simulink model "TenzoDecV3DeltaP"  (Simulink 7.9)
settings: Solver=ode23s  StartTime=0.0  StopTime=15  RelTol=1e-3
values from neighbouring files (symbols this model uses):
  AMI = AK1    [DecV3Vars.m]
  AMin = [ ... (first row only)    [DecV3Vars.m]
  Aoss = AMin-V*ClocalMin    [DecV3Vars.m]
  BMI = BK1    [DecV3Vars.m]
  Bmod = [M BMin]    [DecV3Vars.m]
  Boss = [BMin-V*D V M-V*N]    [DecV3Vars.m]
  ClocalMin = [ ... (first row only)    [DecV3Vars.m]
  CMI = eye(q*mu)    [DecV3Vars.m]
  Coss = eye(n)    [DecV3Vars.m]
  D_phi = [1 1877.59274550691 0]    [DecV3Vars.m]
  D_psi = [1 1877.59274550691 0]    [DecV3Vars.m]
  D_theta = [1 1877.59274550691 0]    [DecV3Vars.m]
  D_thrust = [1 5043.9968441748 6107158.06951568]    [DecV3Vars.m]
  DMI = zeros(q*mu,q)    [DecV3Vars.m]
  Dmod = [N D]    [DecV3Vars.m]
  Doss = zeros(size(Boss))    [DecV3Vars.m]
  EasyHardSat = 0    [DecV3Vars.m]
  F1 = F(:,size(AMin,1)+1:size(F,2))    [DecV3Vars.m]
  F2 = F(:,1:size(AMin,1))    [DecV3Vars.m]
  k1 = 1    [DecV3Vars.m]
  k2 = 1.869    [DecV3Vars.m]
  k3 = 2.002    [DecV3Vars.m]
  k4 = 1.996    [DecV3Vars.m]
  Kt = ct*rho*rp^2*pi()    [DecV3Vars.m]
  Ktm = Km/Kt    [DecV3Vars.m]
  lx = 28.8e-3    (= 0.0288)    [DecV3Vars.m]
  ly = 28.8e-3    (= 0.0288)    [DecV3Vars.m]
  N_phi = [3029.1617545382 41884.8274476077 0]    [DecV3Vars.m]
  N_psi = [3029.1617545382 41884.8274476077 0]    [DecV3Vars.m]
  N_theta = [3029.1617545382 41884.8274476077 0]    [DecV3Vars.m]
  N_thrust = [1073231686.12918 1273486031.3238]    [DecV3Vars.m]
  omega = 0.5    [DecV3Vars.m]
  satMaxRPM = 6000    [DecV3Vars.m]
  satMinRPM = -1300    [DecV3Vars.m]
  satNegThrust = 6    [DecV3Vars.m]
  satTau = 100    [DecV3Vars.m]
  satThrust = 56    [DecV3Vars.m]
  tc = 0.0436    [DecV3Vars.m]
undefined symbols (not defined in the file or in its folder): magnitude, sigbuilder_block
libraries: simulink x6
settings Model: Creator=danilo  LastModifiedBy=userk
settings DebuggingCC: FcnCallInpInsideContextMsg=Use local settings
settings GRTTargetCC: CombineOutputUpdateFcns=off  GRTInterface=on

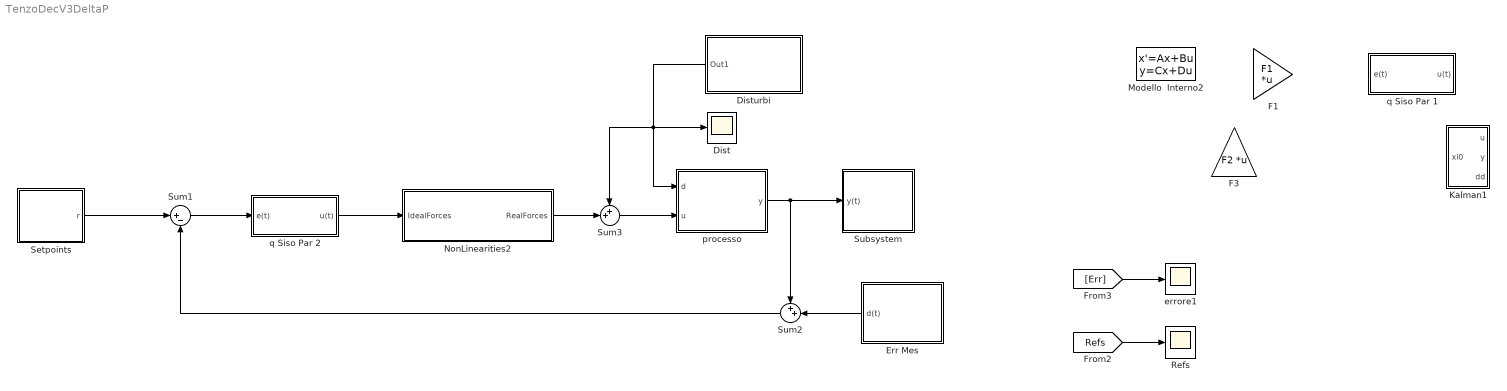
== system TenzoDecV3DeltaP ==
  Dist : Scope
      settings: TimeRange=15  YMin=-0.1  YMax=0.09  SaveName=ScopeData22
  Disturbi : Subsystem
  Err Mes : Subsystem
  F1 : Gain  Gain=F1  Multiplication=Matrix(K*u) (u vector)
  F3 : Gain  Gain=F2  Multiplication=Matrix(K*u) (u vector)
  Kalman1 : Subsystem
  Modello  Interno2 : StateSpace  A=AMI  B=BMI  C=CMI  D=DMI
  NonLinearities2 : Subsystem
  Refs : Scope
  Setpoints : Subsystem
  Subsystem : Subsystem
  Sum1 : Sum  Inputs=|+-
  Sum2 : Sum  Inputs=++|
  Sum3 : Sum  Inputs=++|
  errore1 : Scope
      settings: SaveName=ScopeData8
  processo : Subsystem
  q Siso Par 1 : Subsystem
  q Siso Par 2 : Subsystem
  wires:
  Setpoints/1(r) -> Sum1/1
  processo/1(y) -> Sum2/1, Subsystem/1(y(t))
  Sum1/1 -> q Siso Par 2/1(e(t))
  [Refs] -> Refs/1
  [Err] -> errore1/1
  q Siso Par 2/1(u(t)) -> NonLinearities2/1(IdealForces)
  NonLinearities2/1(RealForces) -> Sum3/2
  Err Mes/1("  d(t)") -> Sum2/2
  Sum2/1 -> Sum1/2
  Disturbi/1(Out1) -> processo/1(d), Dist/1, Sum3/1
  Sum3/1 -> processo/2(u)

== system TenzoDecV3DeltaP/Disturbi ==
  Disturbi Hard : Subsystem
  DisturboEasy : Subsystem
  Manual Switch : simulink/Signal Routing/Manual Switch  sw=0  action=0  varsize=off
  Out1 : Outport
  wires:
  DisturboEasy/1(Out1) -> Manual Switch/1
  Disturbi Hard/1("  d(t)") -> Manual Switch/2
  Manual Switch/1 -> Out1/1

== system TenzoDecV3DeltaP/Err Mes ==
  0.03 sen(80t) : Sin  Amplitude=0.003  Frequency=80  Phase=1  SampleTime=0
  0.2 sen(0.5 t) : Sin  Amplitude=0.02  Frequency=50  Phase=1  SampleTime=0
  Gain : Gain
  Manual Switch1 : simulink/Signal Routing/Manual Switch  sw=0  action=0  varsize=off
  P(s)1 : TransferFcn  Numerator=1  Denominator=[1 9]
  Scope2 : Scope
      settings: SaveName=ScopeData21
  Sum3 : Sum
  Uniform Random Number : UniformRandomNumber  Minimum=-0.05  Maximum=0.05  SampleTime=0.1
  "  d(t)" : Outport
  wires:
  Uniform Random Number/1 -> Sum3/1
  0.2 sen(0.5 t)/1 -> Sum3/2
  Sum3/1 -> P(s)1/1
  0.03 sen(80t)/1 -> Manual Switch1/1
  P(s)1/1 -> Manual Switch1/2
  Gain/1 -> "  d(t)"/1, Scope2/1
  Manual Switch1/1 -> Gain/1

== system TenzoDecV3DeltaP/Kalman1 ==
  u : Inport
  y : Inport  Port=2
  dd : Inport  Port=3
  Mux : Mux  Inputs=[4 4 1]
  filtro di kalman : StateSpace  A=Aoss  B=Boss  C=Coss  D=Doss
  xi0 : Outport
  wires:
  dd/1 -> Mux/3
  y/1 -> Mux/2
  filtro di kalman/1 -> xi0/1
  u/1 -> Mux/1
  Mux/1 -> filtro di kalman/1

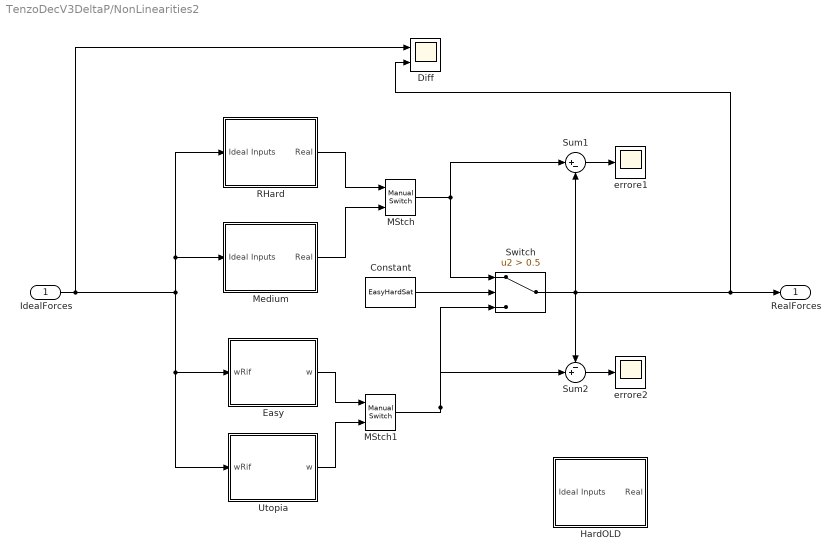
== system TenzoDecV3DeltaP/NonLinearities2 ==
  IdealForces : Inport
  Constant : Constant  Value=EasyHardSat
  Diff : Scope  NumInputPorts=2
      settings: YMin=-37.5~-37.5  YMax=12.5~12.5  SaveName=ScopeData3
  Easy : Subsystem
  HardOLD : Subsystem
  MStch : simulink/Signal Routing/Manual Switch  sw=0  action=0  varsize=off
  MStch1 : simulink/Signal Routing/Manual Switch  sw=1  action=0  varsize=off
  Medium : Subsystem
  RHard : Subsystem
  Sum1 : Sum  Inputs=|+-
  Sum2 : Sum  Inputs=-+|
  Switch : Switch  Criteria=u2 > Threshold  Threshold=0.5
  Utopia : Subsystem
  errore1 : Scope
      settings: SaveName=ScopeData18
  errore2 : Scope
      settings: SaveName=ScopeData20
  RealForces : Outport
  wires:
  Sum2/1 -> errore2/1
  Sum1/1 -> errore1/1
  IdealForces/1 -> Medium/1(Ideal Inputs), RHard/1(Ideal Inputs), Easy/1(wRif), Utopia/1(wRif), Diff/1
  Switch/1 -> Sum2/1, Sum1/2, RealForces/1, Diff/2
  Constant/1 -> Switch/2
  MStch/1 -> Switch/1, Sum1/1
  RHard/1(Real) -> MStch/1
  Medium/1(Real) -> MStch/2
  MStch1/1 -> Switch/3, Sum2/2
  Easy/1(w) -> MStch1/1
  Utopia/1(w) -> MStch1/2

== system TenzoDecV3DeltaP/Setpoints ==
  Mux : Mux  Inputs=[1 1 1 1]
  PsiRef : Step  Time=0.8  After=2.5  SampleTime=0
  Signal Builder : Subsystem  Tag=STV Subsys  LoadFcn=sigbuilder_block('load');  StartFcn=sigbuilder_block('start');  StopFcn=sigbuilder_block('stop');  ClipboardFcn=sigbuilder_block('clipboard');  mask(Sigbuilder block){}
      mask help: Simulink:masks:SigbuilderBlock_MD
      mask init:
      | if ~strcmp(get_param(bdroot(gcbh),'SimulationStatus'),'stopped') tuvar = sigbuilder_block('maskInit'); end
      settings: CopyFcn=sigbuilder_block('copy');  DeleteFcn=sigbuilder_block('delete');  ModelCloseFcn=sigbuilder_block('modelClose');  PreSaveFcn=sigbuilder_block('preSave');  PauseFcn=sigbuilder_block('pause');  ContinueFcn=sigbuilder_block('continue');  NameChangeFcn=sigbuilder_block('namechange');  OpenFcn=sigbuilder_block('open',[357.6 120.8 550.4 400 ]);  CloseFcn=sigbuilder_block('close');
      mask Display: plot(0, 0, 100, 100,[2, 2, 32, 32, 2], [68, 8, 8, 68, 68],[32, 2], [38, 38], [32, 19, 2],[53, 60, 44], [32, 17, 17, 2],[16, 16, 31, 31]);txt = getActiveGroup(gcbh);text(2, 100, txt,'verticalAlignment', 'top');
  ThetRef : Step  Time=0.5  After=2  SampleTime=0
  phiRef : Step  After=1.5  SampleTime=0
  r : Outport
  tag scope: Refs=global
  wires:
  Mux/1 -> r/1, [Refs]
  phiRef/1 -> Mux/1
  ThetRef/1 -> Mux/2
  PsiRef/1 -> Mux/3
  Signal Builder/1(Signal 1) -> Mux/4

== system TenzoDecV3DeltaP/Subsystem ==
  y(t) : Inport
  Output : Subsystem
  uscite : Scope
      settings: TimeRange=15  YMin=-1.4e+10  YMax=6e+09  SaveName=ScopeData2
  wires:
  [Refs] -> Output/2(In2)
  y(t)/1 -> Output/1(In1), uscite/1

== system TenzoDecV3DeltaP/processo ==
  d : Inport
  u : Inport  Port=2
  Mux : Mux  Inputs=[1 4]
  Processo1 : StateSpace  A=AMin  B=Bmod  C=ClocalMin  D=Dmod
  y : Outport
  wires:
  Mux/1 -> Processo1/1
  d/1 -> Mux/1
  Processo1/1 -> y/1
  u/1 -> Mux/2

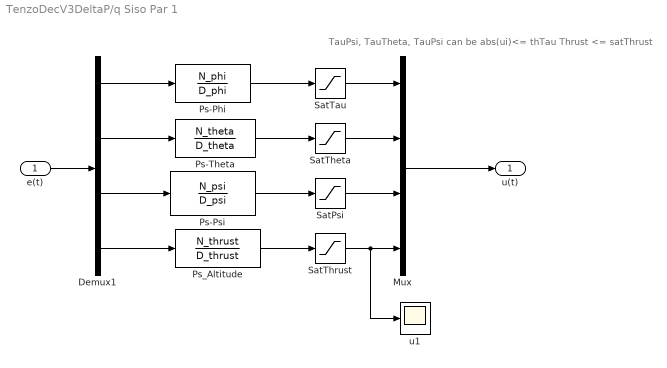
== system TenzoDecV3DeltaP/q Siso Par 1 ==
  note: TauPsi, TauTheta, TauPsi
      |  can be abs(ui)<= thTau
      | Thrust <= satThrust
  e(t) : Inport
  Demux1 : Demux
  Mux : Mux
  Ps-Phi : TransferFcn  Numerator=N_phi  Denominator=D_phi
  Ps-Psi : TransferFcn  Numerator=N_psi  Denominator=D_psi
  Ps-Theta : TransferFcn  Numerator=N_theta  Denominator=D_theta
  Ps_Altitude : TransferFcn  Numerator=N_thrust  Denominator=D_thrust
  SatPsi : Saturate  UpperLimit=satTau  LowerLimit=-satTau
  SatTau : Saturate  UpperLimit=satTau  LowerLimit=-satTau
  SatTheta : Saturate  UpperLimit=satTau  LowerLimit=-satTau
  SatThrust : Saturate  UpperLimit=satThrust  LowerLimit=-satNegThrust
  u1 : Scope
      settings: SaveName=ScopeData9
  u(t) : Outport
  wires:
  SatTau/1 -> Mux/1
  SatTheta/1 -> Mux/2
  SatPsi/1 -> Mux/3
  SatThrust/1 -> u1/1, Mux/4
  Demux1/1 -> Ps-Phi/1
  Demux1/3 -> Ps-Psi/1
  Demux1/4 -> Ps_Altitude/1
  Ps-Phi/1 -> SatTau/1
  Ps_Altitude/1 -> SatThrust/1
  Demux1/2 -> Ps-Theta/1
  Ps-Theta/1 -> SatTheta/1
  Ps-Psi/1 -> SatPsi/1
  e(t)/1 -> Demux1/1
  Mux/1 -> u(t)/1

== system TenzoDecV3DeltaP/q Siso Par 2 ==
  note: TauPsi, TauTheta, TauPsi
      |  can be abs(ui)<= thTau
      | Thrust <= satThrust
  e(t) : Inport
  Demux1 : Demux
  Mux : Mux
  Old q SISO + sat : Subsystem
  Ps-Phi : TransferFcn  Numerator=N_phi  Denominator=D_phi
  Ps-Psi : TransferFcn  Numerator=N_psi  Denominator=D_psi
  Ps-Theta : TransferFcn  Numerator=N_theta  Denominator=D_theta
  Ps_Altitude : TransferFcn  Numerator=N_thrust  Denominator=D_thrust
  To Workspace : ToWorkspace  VariableName=simout  SampleTime=-1  SaveFormat=Structure
  u1 : Scope
      settings: YMin=-8e+08  YMax=5e+07  SaveName=ScopeData9
  u(t) : Outport
  wires:
  Mux/1 -> u(t)/1
  e(t)/1 -> Demux1/1, To Workspace/1, [Err]
  Ps-Psi/1 -> Mux/3
  Ps-Theta/1 -> Mux/2
  Demux1/2 -> Ps-Theta/1
  Ps_Altitude/1 -> Mux/4, u1/1
  Ps-Phi/1 -> Mux/1
  Demux1/4 -> Ps_Altitude/1
  Demux1/3 -> Ps-Psi/1
  Demux1/1 -> Ps-Phi/1

== system TenzoDecV3DeltaP/Disturbi/Disturbi Hard ==
  0.2 sen(0.5 t) : Sin  Amplitude=0.2  Frequency=0.5  Phase=1  SampleTime=0
  0.2 sen(0.5 t)1 : Sin  Amplitude=0.1  Frequency=1.5  Phase=1.5  SampleTime=0
  0.5sen(0.5 t) : Sin  Amplitude=0.5  Frequency=0.5  Phase=1  SampleTime=0
  Manual Switch1 : simulink/Signal Routing/Manual Switch  sw=0  action=0  varsize=off
  P(s)1 : TransferFcn  Numerator=1  Denominator=[1 4]
  Sum3 : Sum  Inputs=+++
  Uniform Random Number : UniformRandomNumber  Minimum=-0.5  Maximum=0.5  SampleTime=0.1
  d(t) : Gain
  d(t) raw : Scope
      settings: TimeRange=15  YMin=-0.65  YMax=0.05  SaveName=ScopeData24
  "  d(t)" : Outport
  wires:
  Uniform Random Number/1 -> Sum3/1
  0.2 sen(0.5 t)/1 -> Sum3/3
  Sum3/1 -> P(s)1/1, d(t) raw/1
  0.5sen(0.5 t)/1 -> Manual Switch1/1
  P(s)1/1 -> Manual Switch1/2
  d(t)/1 -> "  d(t)"/1
  Manual Switch1/1 -> d(t)/1
  0.2 sen(0.5 t)1/1 -> Sum3/2

== system TenzoDecV3DeltaP/Disturbi/DisturboEasy ==
  Clock : Clock
  Constant : Constant  Value=0
  Constant1 : Constant  Value=0
  Manual Switch : simulink/Signal Routing/Manual Switch  sw=0  action=0  varsize=off
  Switch : Switch  Threshold=5
  dist : Scope
      settings: SaveName=ScopeData5
  disturbo : Subsystem
  Out1 : Outport
  wires:
  Clock/1 -> Switch/2
  disturbo/1(d) -> Switch/1
  Constant/1 -> Switch/3
  Constant1/1 -> Manual Switch/1
  Switch/1 -> Manual Switch/2
  Manual Switch/1 -> dist/1, Out1/1

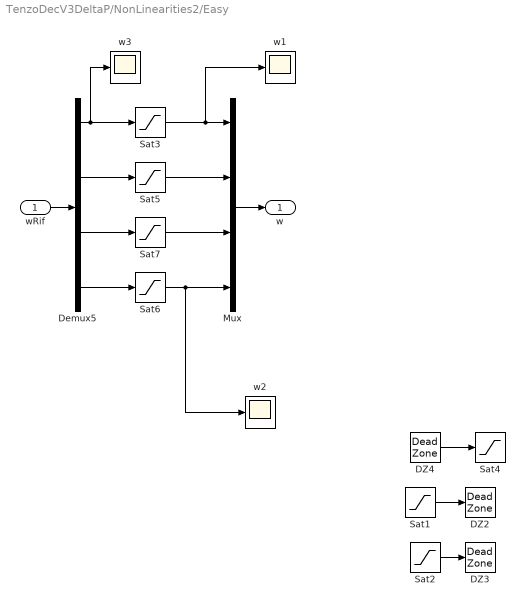
== system TenzoDecV3DeltaP/NonLinearities2/Easy ==
  wRif : Inport
  DZ2 : DeadZone  LowerValue=0  UpperValue=deadMotorsZone  SaturateOnIntegerOverflow=on
  DZ3 : DeadZone  LowerValue=0  UpperValue=deadMotorsZone  SaturateOnIntegerOverflow=on
  DZ4 : DeadZone  LowerValue=0  UpperValue=deadMotorsZone  SaturateOnIntegerOverflow=on
  Demux5 : Demux
  Mux : Mux
  Sat1 : Saturate  UpperLimit=satMaxRPM  LowerLimit=0
  Sat2 : Saturate  UpperLimit=satMaxRPM  LowerLimit=0
  Sat3 : Saturate  UpperLimit=satTau  LowerLimit=-satTau
  Sat4 : Saturate  UpperLimit=satMaxRPM  LowerLimit=0
  Sat5 : Saturate  UpperLimit=satTau  LowerLimit=-satTau
  Sat6 : Saturate  UpperLimit=satThrust  LowerLimit=-satNegThrust
  Sat7 : Saturate  UpperLimit=satTau  LowerLimit=-satTau
  w1 : Scope
      settings: YMin=-1.5e+42  YMax=2.25e+42  SaveName=ScopeData15
  w2 : Scope
      settings: YMin=-8e+50  YMax=5e+50  SaveName=ScopeData10
  w3 : Scope
      settings: YMin=904.495  YMax=999.705  SaveName=ScopeData16
  w : Outport
  wires:
  Demux5/4 -> Sat6/1
  Demux5/3 -> Sat7/1
  Demux5/2 -> Sat5/1
  Sat7/1 -> Mux/3
  Sat6/1 -> w2/1, Mux/4
  Sat5/1 -> Mux/2
  Sat3/1 -> Mux/1, w1/1
  Demux5/1 -> Sat3/1, w3/1
  wRif/1 -> Demux5/1
  Mux/1 -> w/1
  DZ4/1 -> Sat4/1
  Sat1/1 -> DZ2/1
  Sat2/1 -> DZ3/1

== system TenzoDecV3DeltaP/NonLinearities2/HardOLD ==
  Ideal Inputs : Inport
  Demux11 : Demux
  Motors : Subsystem
  Mux3 : Mux
  T*toW : MATLAB Function  TreatAsAtomicUnit=on
  WtoTreal : Subsystem
  ideal : Scope
      settings: YMin=-5e+71  YMax=4e+71  SaveName=ScopeData25
  real : Scope
      settings: YMin=-2.5e+113  YMax=4.25e+114  SaveName=ScopeData26
  wReal : Scope
      settings: SaveName=ScopeData27
  wideal : Scope
      settings: YMin=-4.5e+73  YMax=4.5e+73  SaveName=ScopeData23
  Real : Outport
  wires:
  WtoTreal/1(U(t)) -> real/1, Real/1
  Ideal Inputs/1 -> ideal/1, Demux11/1
  Mux3/1 -> wideal/1, Motors/1(wRif)
  Motors/1(w) -> wReal/1, WtoTreal/1(w(t))
  Demux11/1 -> T*toW/1(taux)
  Demux11/2 -> T*toW/2(tauy)
  Demux11/3 -> T*toW/3(tauz)
  Demux11/4 -> T*toW/4(Thrust)
  T*toW/1(w1) -> Mux3/1
  T*toW/2(w2) -> Mux3/2
  T*toW/3(w3) -> Mux3/3
  T*toW/4(w4) -> Mux3/4

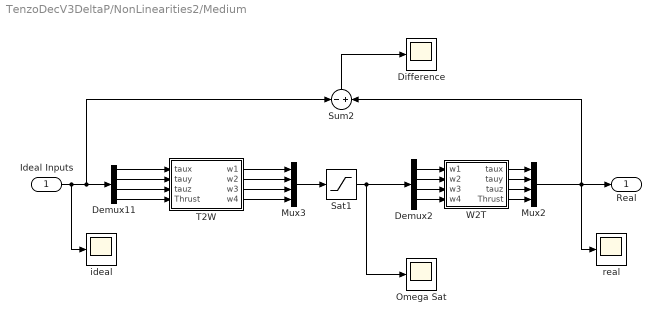
== system TenzoDecV3DeltaP/NonLinearities2/Medium ==
  Ideal Inputs : Inport
  Demux11 : Demux
  Demux2 : Demux
  Difference : Scope
      settings: YMin=-4e-08  YMax=1.2e-07  SaveName=ScopeData28
  Mux2 : Mux
  Mux3 : Mux
  Omega Sat : Scope
      settings: YMin=-6000  YMax=6000  SaveName=ScopeData29
  Sat1 : Saturate  UpperLimit=8000  LowerLimit=-10000
  Sum2 : Sum  Inputs=-+
  T2W : MATLAB Function  TreatAsAtomicUnit=on
  W2T : MATLAB Function  TreatAsAtomicUnit=on
  ideal : Scope
      settings: YMin=-5e+71  YMax=4e+71  SaveName=ScopeData25
  real : Scope
      settings: YMin=-2.5e+113  YMax=4.25e+114  SaveName=ScopeData26
  Real : Outport
  wires:
  T2W/4(w4) -> Mux3/4
  T2W/3(w3) -> Mux3/3
  T2W/2(w2) -> Mux3/2
  T2W/1(w1) -> Mux3/1
  Demux11/4 -> T2W/4(Thrust)
  Demux11/3 -> T2W/3(tauz)
  Demux11/2 -> T2W/2(tauy)
  Demux11/1 -> T2W/1(taux)
  Mux3/1 -> Sat1/1
  Ideal Inputs/1 -> ideal/1, Demux11/1, Sum2/1
  Mux2/1 -> real/1, Real/1, Sum2/2
  Demux2/1 -> W2T/1(w1)
  Demux2/2 -> W2T/2(w2)
  Demux2/3 -> W2T/3(w3)
  Demux2/4 -> W2T/4(w4)
  W2T/1(taux) -> Mux2/1
  W2T/2(tauy) -> Mux2/2
  W2T/3(tauz) -> Mux2/3
  W2T/4(Thrust) -> Mux2/4
  Sum2/1 -> Difference/1
  Sat1/1 -> Demux2/1, Omega Sat/1

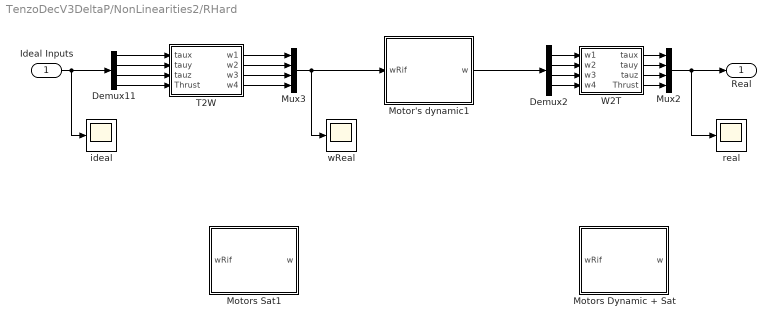
== system TenzoDecV3DeltaP/NonLinearities2/RHard ==
  Ideal Inputs : Inport
  Demux11 : Demux
  Demux2 : Demux
  Motor's dynamic1 : Subsystem
  Motors Dynamic + Sat : Subsystem
  Motors Sat1 : Subsystem
  Mux2 : Mux
  Mux3 : Mux
  T2W : MATLAB Function  TreatAsAtomicUnit=on
  W2T : MATLAB Function  TreatAsAtomicUnit=on
  ideal : Scope
      settings: YMin=-5e+71  YMax=4e+71  SaveName=ScopeData25
  real : Scope
      settings: YMin=-2.5e+113  YMax=4.25e+114  SaveName=ScopeData26
  wReal : Scope
      settings: YMin=-7500  YMax=35000  SaveName=ScopeData27
  Real : Outport
  wires:
  W2T/4(Thrust) -> Mux2/4
  W2T/3(tauz) -> Mux2/3
  W2T/2(tauy) -> Mux2/2
  W2T/1(taux) -> Mux2/1
  Demux2/4 -> W2T/4(w4)
  Demux2/3 -> W2T/3(w3)
  Demux2/2 -> W2T/2(w2)
  Demux2/1 -> W2T/1(w1)
  Mux2/1 -> Real/1, real/1
  Ideal Inputs/1 -> Demux11/1, ideal/1
  Mux3/1 -> wReal/1, Motor's dynamic1/1(wRif)
  Demux11/1 -> T2W/1(taux)
  Demux11/2 -> T2W/2(tauy)
  Demux11/3 -> T2W/3(tauz)
  Demux11/4 -> T2W/4(Thrust)
  T2W/1(w1) -> Mux3/1
  T2W/2(w2) -> Mux3/2
  T2W/3(w3) -> Mux3/3
  T2W/4(w4) -> Mux3/4
  Motor's dynamic1/1(w) -> Demux2/1

== system TenzoDecV3DeltaP/NonLinearities2/Utopia ==
  wRif : Inport
  DZ3 : DeadZone  LowerValue=0  UpperValue=deadMotorsZone  SaturateOnIntegerOverflow=on
  Demux5 : Demux
  Mux : Mux
  Sat2 : Saturate  UpperLimit=satMaxRPM  LowerLimit=0
  w : Outport
  wires:
  Sat2/1 -> DZ3/1
  ? -> ?
  Mux/1 -> w/1
  wRif/1 -> Demux5/1
  Demux5/1 -> Mux/1
  Demux5/2 -> Mux/2
  Demux5/3 -> Mux/3
  Demux5/4 -> Mux/4

== system TenzoDecV3DeltaP/Setpoints/Signal Builder ==
  Demux : Demux  Tag=STV Demux  Outputs=1
  FromWs : FromWorkspace  Tag=STV FromWs  VariableName=tuvar  SampleTime=0  SigBuilderData=DataTag0  VnvData=DataTag1
      SigBuilderData=|
      | common.afterFinalStr = 'Extrapolate'
      | common.sampleTime = 0
      | dataSet.timeRange = [0 10]
      | dataSet.name = 'Group 1'
      | sbobj.Groups.Name = 'Group 1'
      | sbobj.Groups.Signals.Name = 'Signal 1'
      | sbobj.Groups.Signals.XData = [0 4.06 6 6 10]
      | sbobj.Groups.Signals.YData = [-2.77555756156e-17 1 1 0.995 0.795]
  Signal 1 : Outport  Tag=STV Outport
  wires:
  Demux/1 -> Signal 1/1
  FromWs/1 -> Demux/1

== system TenzoDecV3DeltaP/Subsystem/Output ==
  In1 : Inport
  In2 : Inport  Port=2
  Demux1 : Demux
  Demux2 : Demux
  Mux{2..5} (4 alike) : Mux  Inputs=2
  uscite{,1..3} (4 alike) : Scope
      uscite settings: TickLabels=on  YMin=1.495  YMax=1.5065
      uscite1 settings: TickLabels=on  TimeRange=30  YMin=0.75  YMax=4.25  SaveName=ScopeData4
      uscite2 settings: TickLabels=on  TimeRange=15  YMin=-1.75e+15  YMax=1.75e+15  SaveName=ScopeData6
      uscite3 settings: TickLabels=on  YMin=0  YMax=1.05  SaveName=ScopeData7
  wires:
  Demux1/1 -> Mux3/2
  In2/1 -> Demux1/1
  In1/1 -> Demux2/1
  Mux3/1 -> uscite/1
  Demux2/1 -> Mux3/1
  Mux2/1 -> uscite1/1
  Demux2/2 -> Mux2/1
  Mux4/1 -> uscite2/1
  Demux2/3 -> Mux4/1
  Mux5/1 -> uscite3/1
  Demux2/4 -> Mux5/1
  Demux1/2 -> Mux2/2
  Demux1/3 -> Mux4/2
  Demux1/4 -> Mux5/2

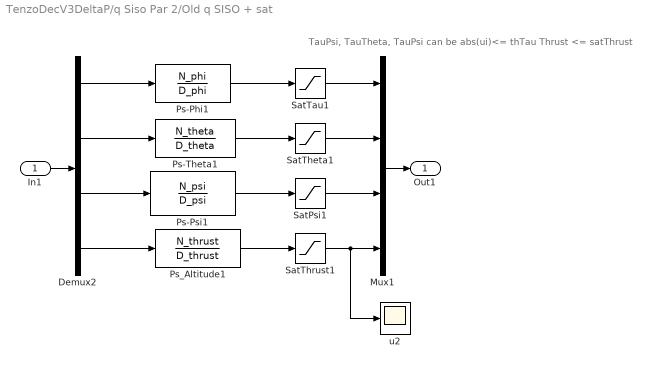
== system TenzoDecV3DeltaP/q Siso Par 2/Old q SISO + sat ==
  note: TauPsi, TauTheta, TauPsi
      |  can be abs(ui)<= thTau
      | Thrust <= satThrust
  In1 : Inport
  Demux2 : Demux
  Mux1 : Mux
  Ps-Phi1 : TransferFcn  Numerator=N_phi  Denominator=D_phi
  Ps-Psi1 : TransferFcn  Numerator=N_psi  Denominator=D_psi
  Ps-Theta1 : TransferFcn  Numerator=N_theta  Denominator=D_theta
  Ps_Altitude1 : TransferFcn  Numerator=N_thrust  Denominator=D_thrust
  SatPsi1 : Saturate  UpperLimit=satTau  LowerLimit=-satTau
  SatTau1 : Saturate  UpperLimit=satTau  LowerLimit=-satTau
  SatTheta1 : Saturate  UpperLimit=satTau  LowerLimit=-satTau
  SatThrust1 : Saturate  UpperLimit=satThrust  LowerLimit=-satNegThrust
  u2 : Scope
      settings: SaveName=ScopeData12
  Out1 : Outport
  wires:
  Ps-Psi1/1 -> SatPsi1/1
  Ps-Theta1/1 -> SatTheta1/1
  Demux2/2 -> Ps-Theta1/1
  Ps_Altitude1/1 -> SatThrust1/1
  Ps-Phi1/1 -> SatTau1/1
  Demux2/4 -> Ps_Altitude1/1
  Demux2/3 -> Ps-Psi1/1
  Demux2/1 -> Ps-Phi1/1
  SatThrust1/1 -> Mux1/4, u2/1
  SatPsi1/1 -> Mux1/3
  SatTheta1/1 -> Mux1/2
  SatTau1/1 -> Mux1/1
  In1/1 -> Demux2/1
  Mux1/1 -> Out1/1

== system TenzoDecV3DeltaP/Disturbi/DisturboEasy/disturbo ==
  Constant : Constant
  Sine Wave : Sin  Amplitude=0.5  Frequency=omega  SampleTime=0
  Sum2 : Sum  Inputs=|++
  d : Outport
  wires:
  Sine Wave/1 -> Sum2/2
  Constant/1 -> Sum2/1
  Sum2/1 -> d/1

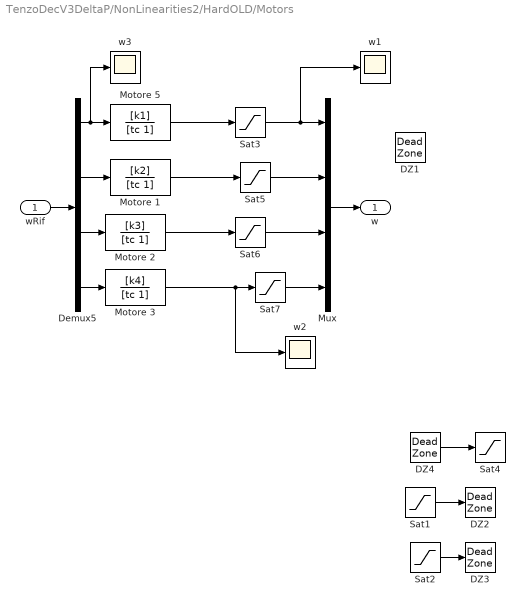
== system TenzoDecV3DeltaP/NonLinearities2/HardOLD/Motors ==
  wRif : Inport
  DZ{1..4} (4 alike) : DeadZone  LowerValue=0  UpperValue=deadMotorsZone  SaturateOnIntegerOverflow=on
  Demux5 : Demux
  Motore 1 : TransferFcn  Numerator=[k2]  Denominator=[tc 1]
  Motore 2 : TransferFcn  Numerator=[k3]  Denominator=[tc 1]
  Motore 3 : TransferFcn  Numerator=[k4]  Denominator=[tc 1]
  Motore 5 : TransferFcn  Numerator=[k1]  Denominator=[tc 1]
  Mux : Mux
  Sat1 : Saturate  UpperLimit=satMaxRPM  LowerLimit=0
  Sat2 : Saturate  UpperLimit=satMaxRPM  LowerLimit=0
  Sat{3,5..7} (4 alike) : Saturate  UpperLimit=satMaxRPM  LowerLimit=satMinRPM
  Sat4 : Saturate  UpperLimit=satMaxRPM  LowerLimit=0
  w1 : Scope
      settings: YMin=-1.5e+42  YMax=2.25e+42  SaveName=ScopeData15
  w2 : Scope
      settings: YMin=-8e+50  YMax=5e+50  SaveName=ScopeData10
  w3 : Scope
      settings: YMin=904.495  YMax=999.705  SaveName=ScopeData16
  w : Outport
  wires:
  Sat7/1 -> Mux/4
  Sat6/1 -> Mux/3
  Sat5/1 -> Mux/2
  Sat3/1 -> w1/1, Mux/1
  Sat2/1 -> DZ3/1
  Sat1/1 -> DZ2/1
  DZ4/1 -> Sat4/1
  Motore 3/1 -> Sat7/1, w2/1
  Motore 2/1 -> Sat6/1
  Motore 1/1 -> Sat5/1
  Motore 5/1 -> Sat3/1
  Mux/1 -> w/1
  wRif/1 -> Demux5/1
  Demux5/4 -> Motore 3/1
  Demux5/3 -> Motore 2/1
  Demux5/2 -> Motore 1/1
  Demux5/1 -> w3/1, Motore 5/1

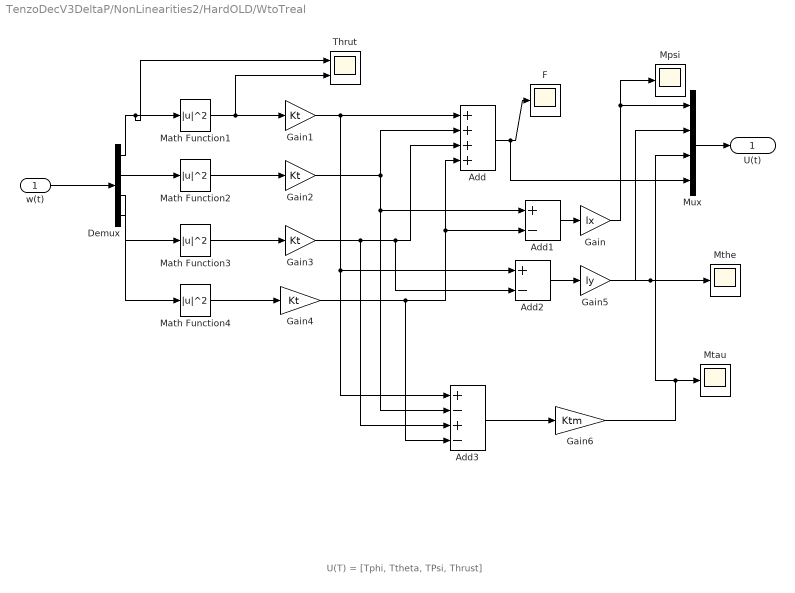
== system TenzoDecV3DeltaP/NonLinearities2/HardOLD/WtoTreal ==
  note: U(T) = [Tphi, Ttheta, TPsi, Thrust]
  w(t) : Inport
  Add : Sum  Inputs=++++
  Add1 : Sum  Inputs=+-
  Add2 : Sum  Inputs=+-
  Add3 : Sum  Inputs=+-+-
  Demux : Demux
  F : Scope
      settings: SaveName=ScopeData17
  Gain : Gain  Gain=lx
  Gain{1..4} (4 alike) : Gain  Gain=Kt
  Gain5 : Gain  Gain=ly
  Gain6 : Gain  Gain=Ktm
  Math Function{1..4} (4 alike) : Math  Operator=magnitude^2  SaturateOnIntegerOverflow=on
  Mpsi : Scope
      settings: SaveName=ScopeData14
  Mtau : Scope
      settings: SaveName=ScopeData11
  Mthe : Scope
      settings: SaveName=ScopeData13
  Mux : Mux
  Thrut : Scope  NumInputPorts=2
      settings: YMin=-5~-5  YMax=5~5  SaveName=ScopeData19
  U(t) : Outport
  wires:
  Math Function1/1 -> Gain1/1, Thrut/2
  Math Function2/1 -> Gain2/1
  Math Function3/1 -> Gain3/1
  Math Function4/1 -> Gain4/1
  Gain1/1 -> Add/1, Add2/1, Add3/1
  Gain2/1 -> Add/2, Add1/1, Add3/2
  Gain3/1 -> Add/3, Add2/2, Add3/3
  Gain4/1 -> Add/4, Add1/2, Add3/4
  Add/1 -> Mux/4, F/1
  Add1/1 -> Gain/1
  Add2/1 -> Gain5/1
  Gain/1 -> Mux/1, Mpsi/1
  Gain5/1 -> Mux/2, Mthe/1
  Add3/1 -> Gain6/1
  Gain6/1 -> Mux/3, Mtau/1
  Demux/1 -> Math Function1/1, Thrut/1
  Demux/2 -> Math Function2/1
  Mux/1 -> U(t)/1
  Demux/3 -> Math Function3/1
  Demux/4 -> Math Function4/1
  w(t)/1 -> Demux/1

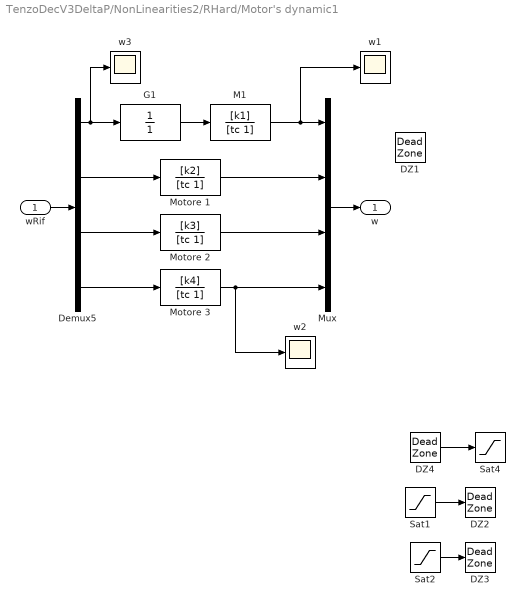
== system TenzoDecV3DeltaP/NonLinearities2/RHard/Motor's dynamic1 ==
  wRif : Inport
  DZ{1..4} (4 alike) : DeadZone  LowerValue=0  UpperValue=deadMotorsZone  SaturateOnIntegerOverflow=on
  Demux5 : Demux
  G1 : TransferFcn  Denominator=[1]
  M1 : TransferFcn  Numerator=[k1]  Denominator=[tc 1]
  Motore 1 : TransferFcn  Numerator=[k2]  Denominator=[tc 1]
  Motore 2 : TransferFcn  Numerator=[k3]  Denominator=[tc 1]
  Motore 3 : TransferFcn  Numerator=[k4]  Denominator=[tc 1]
  Mux : Mux
  Sat1 : Saturate  UpperLimit=satMaxRPM  LowerLimit=0
  Sat2 : Saturate  UpperLimit=satMaxRPM  LowerLimit=0
  Sat4 : Saturate  UpperLimit=satMaxRPM  LowerLimit=0
  w1 : Scope
      settings: YMin=-2250  YMax=3500  SaveName=ScopeData15
  w2 : Scope
      settings: YMin=-8e+50  YMax=5e+50  SaveName=ScopeData10
  w3 : Scope
      settings: YMin=-45000  YMax=60000  SaveName=ScopeData16
  w : Outport
  wires:
  Sat2/1 -> DZ3/1
  Sat1/1 -> DZ2/1
  DZ4/1 -> Sat4/1
  Motore 3/1 -> Mux/4, w2/1
  Motore 2/1 -> Mux/3
  Motore 1/1 -> Mux/2
  G1/1 -> M1/1
  Mux/1 -> w/1
  wRif/1 -> Demux5/1
  Demux5/4 -> Motore 3/1
  Demux5/3 -> Motore 2/1
  Demux5/2 -> Motore 1/1
  Demux5/1 -> w3/1, G1/1
  M1/1 -> w1/1, Mux/1

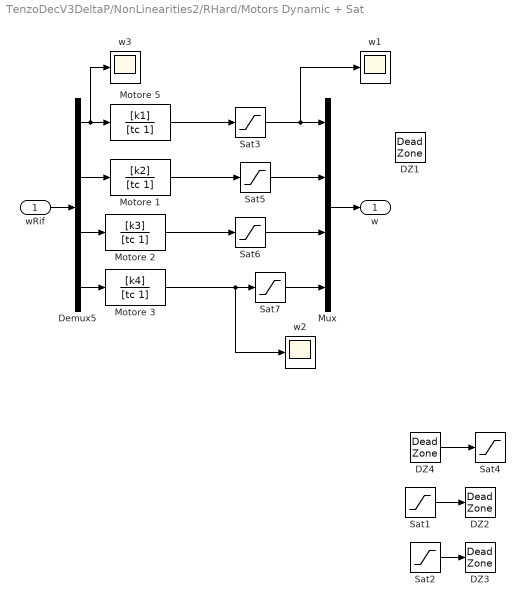
== system TenzoDecV3DeltaP/NonLinearities2/RHard/Motors Dynamic + Sat ==
  wRif : Inport
  DZ{1..4} (4 alike) : DeadZone  LowerValue=0  UpperValue=deadMotorsZone  SaturateOnIntegerOverflow=on
  Demux5 : Demux
  Motore 1 : TransferFcn  Numerator=[k2]  Denominator=[tc 1]
  Motore 2 : TransferFcn  Numerator=[k3]  Denominator=[tc 1]
  Motore 3 : TransferFcn  Numerator=[k4]  Denominator=[tc 1]
  Motore 5 : TransferFcn  Numerator=[k1]  Denominator=[tc 1]
  Mux : Mux
  Sat1 : Saturate  UpperLimit=satMaxRPM  LowerLimit=0
  Sat2 : Saturate  UpperLimit=satMaxRPM  LowerLimit=0
  Sat{3,5..7} (4 alike) : Saturate  UpperLimit=satMaxRPM  LowerLimit=satMinRPM
  Sat4 : Saturate  UpperLimit=satMaxRPM  LowerLimit=0
  w1 : Scope
      settings: YMin=-1.5e+42  YMax=2.25e+42  SaveName=ScopeData15
  w2 : Scope
      settings: YMin=-8e+50  YMax=5e+50  SaveName=ScopeData10
  w3 : Scope
      settings: YMin=904.495  YMax=999.705  SaveName=ScopeData16
  w : Outport
  wires:
  Sat7/1 -> Mux/4
  Sat6/1 -> Mux/3
  Sat5/1 -> Mux/2
  Sat3/1 -> w1/1, Mux/1
  Sat2/1 -> DZ3/1
  Sat1/1 -> DZ2/1
  DZ4/1 -> Sat4/1
  Motore 3/1 -> Sat7/1, w2/1
  Motore 2/1 -> Sat6/1
  Motore 1/1 -> Sat5/1
  Motore 5/1 -> Sat3/1
  Mux/1 -> w/1
  wRif/1 -> Demux5/1
  Demux5/4 -> Motore 3/1
  Demux5/3 -> Motore 2/1
  Demux5/2 -> Motore 1/1
  Demux5/1 -> w3/1, Motore 5/1

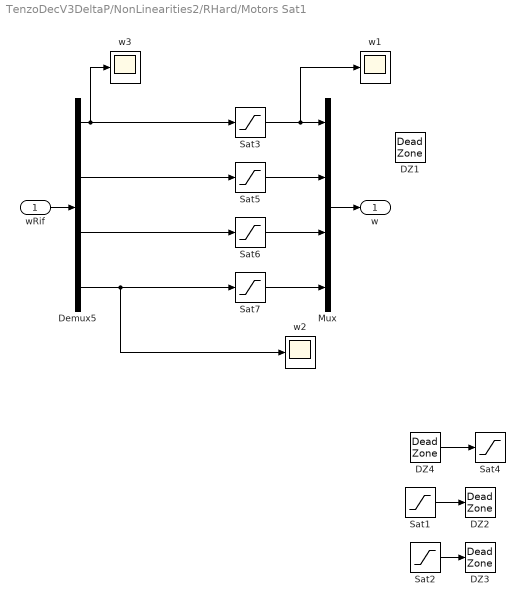
== system TenzoDecV3DeltaP/NonLinearities2/RHard/Motors Sat1 ==
  wRif : Inport
  DZ{1..4} (4 alike) : DeadZone  LowerValue=0  UpperValue=deadMotorsZone  SaturateOnIntegerOverflow=on
  Demux5 : Demux
  Mux : Mux
  Sat1 : Saturate  UpperLimit=satMaxRPM  LowerLimit=0
  Sat2 : Saturate  UpperLimit=satMaxRPM  LowerLimit=0
  Sat{3,5..7} (4 alike) : Saturate  UpperLimit=satMaxRPM  LowerLimit=satMinRPM
  Sat4 : Saturate  UpperLimit=satMaxRPM  LowerLimit=0
  w1 : Scope
      settings: YMin=-1.5e+42  YMax=2.25e+42  SaveName=ScopeData15
  w2 : Scope
      settings: YMin=-8e+50  YMax=5e+50  SaveName=ScopeData10
  w3 : Scope
      settings: YMin=904.495  YMax=999.705  SaveName=ScopeData16
  w : Outport
  wires:
  Sat7/1 -> Mux/4
  Sat6/1 -> Mux/3
  Sat5/1 -> Mux/2
  Sat3/1 -> w1/1, Mux/1
  Sat2/1 -> DZ3/1
  Sat1/1 -> DZ2/1
  DZ4/1 -> Sat4/1
  Mux/1 -> w/1
  wRif/1 -> Demux5/1
  Demux5/4 -> Sat7/1, w2/1
  Demux5/3 -> Sat6/1
  Demux5/2 -> Sat5/1
  Demux5/1 -> w3/1, Sat3/1

== matlab function NonLinearities2/HardOLD/T*toW ==
  data: taux input double; tauy input double; tauz input double; Thrust input double; w1 output double; w2 output double; w3 output double; w4 output double
function [w1,w2,w3,w4] = mixer(taux,tauy,tauz,Thrust)
%#codegen
%% Physical properties of the environment
g=9.81; %Acceleration of gravity (m)
rho=1.2; %Density of air (m^3.kg^-1)

%% Physical properties of the quadrotor

% Total mass of the quadrotor [Kg]
mq=0.82;
% Motor length along x-axis (m). All motors have equal sizes.
lx=28.8e-3;
% Motor length along y-axis (m)
ly=28.8e-3;
% Motor length along z-axis (m)
lz=26e-3;

% Distance from the center of gravity to the center of a motor (m).
% The quadrotor is symmetric regarding the XZ and YZ planes, so
% dcg is the same for all motors.
dcg=0.288; 


% Inflow coefficient
If = -0.3559;

% Thrust coefficient of the propeller and Power coefficient
cp=0.0743; 
ct=0.1154;

% Propeller radius (m)
rp=25.4e-3; 
% Constant value to calculate the moment provided
% by a propeller given its angular speed (kg.m^2.rad^-1)
Km=cp*4*rho*rp^5/pi()^3; 
% Constant value to calculate the thrust provided
% by a propeller given its angular speed (kg.m.rad^-1) 
%Kt=ct*4*rho*rp^4/pi()^2; 
Kt=ct*rho*rp^2*pi();
% Constant that relates thrust and moment of a propeller.
Ktm=Km/Kt;
k1=2.028; %Transfer-function gain of motor 1
k2=1.869; %Transfer-function gain of motor 2
k3=2.002; %Transfer-function gain of motor 3
k4=1.996; %Transfer-function gain of motor 4
tc=0.00436; %Time-constant of the motors (assumed equal for all motors) 0.436

dz1=1247.4; %PWM dead-zone of motor 1 given its first-order transfer
% function (micro-seconds)
dz2=1247.8; % PWM dead-zone of motor 2 given its first-order transfer
%function (micro-seconds)
dz3=1246.4; % PWM dead-zone of motor 3 given its first-order transfer
%function (micro-seconds)
dz4=1247.9; % PWM dead-zone of motor 4 given its first-order transfer
% 
% g_m1=tf(k1,[tc 1]); % First-order transfer-function of motor 1
% g_m2=tf(k2,[tc 1]); % First-order transfer-function of motor 2
% g_m3=tf(k3,[tc 1]); % First-order transfer-function of motor 3
% g_m4=tf(k4,[tc 1]); % First-order transfer-function of motor 4

%vNote: If the behavior of the motors is not linear, linearization around
% an operating point is required to attain these transfer-functions.
PWM_max=2200; %Upper limit of the PWM signal provided to
%the motors (micro-seconds)
w0c=sqrt(g*mq/Kt);
%X0c=w0c;
Ft0=mq*g;


%% u=[T; taux; tauy; tauz];

% WTF = [ -Kt -Kt -Kt -Kt;
%          0   -lx*Kt  0  lx*Kt;
%         ly*Kt  0  -ly*Kt  0;
%         Ktm -Ktm Ktm -Ktm];   
%    T= WTF^(-1)*[Thrust; taux; tauy; tauz];

%%  u=[taux; tauy; tauz, T];

WTF = [     0   -lx*Kt  0  lx*Kt;
            ly*Kt  0  -ly*Kt  0;
            Ktm -Ktm Ktm -Ktm;
            -Kt -Kt -Kt -Kt];  
T= WTF\[taux; tauy; tauz; Thrust];

%% Conversion

    w1 = T(1);
    w2 = T(2);
    w3 = T(3);
    w4 = T(4);

== matlab function NonLinearities2/Medium/T2W ==
  data: taux input double; tauy input double; tauz input double; Thrust input double; w1 output double; w2 output double; w3 output double; w4 output double
function [w1,w2,w3,w4] = mixer(taux,tauy,tauz,Thrust)
%#codegen
%% Physical properties of the environment
g=9.81; %Acceleration of gravity (m)
rho=1.2; %Density of air (m^3.kg^-1)

%% Physical properties of the quadrotor

% Total mass of the quadrotor [Kg]
mq=0.82;
% Motor length along x-axis (m). All motors have equal sizes.
lx=28.8e-3;
% Motor length along y-axis (m)
ly=28.8e-3;
% Motor length along z-axis (m)
lz=26e-3;

% Distance from the center of gravity to the center of a motor (m).
% The quadrotor is symmetric regarding the XZ and YZ planes, so
% dcg is the same for all motors.
dcg=0.288; 


% Inflow coefficient
If = -0.3559;

% Thrust coefficient of the propeller and Power coefficient
cp=0.0743; 
ct=0.1154;

% Propeller radius (m)
rp=25.4e-3; 
% Constant value to calculate the moment provided
% by a propeller given its angular speed (kg.m^2.rad^-1)
Km=cp*4*rho*rp^5/pi()^3; 
% Constant value to calculate the thrust provided
% by a propeller given its angular speed (kg.m.rad^-1) 
%Kt=ct*4*rho*rp^4/pi()^2; 
Kt=ct*rho*rp^4*pi();
% Constant that relates thrust and moment of a propeller.
Ktm=Km/Kt;
k1=2.028; %Transfer-function gain of motor 1
k2=1.869; %Transfer-function gain of motor 2
k3=2.002; %Transfer-function gain of motor 3
k4=1.996; %Transfer-function gain of motor 4
tc=0.00436; %Time-constant of the motors (assumed equal for all motors) 0.436

dz1=1247.4; %PWM dead-zone of motor 1 given its first-order transfer
% function (micro-seconds)
dz2=1247.8; % PWM dead-zone of motor 2 given its first-order transfer
%function (micro-seconds)
dz3=1246.4; % PWM dead-zone of motor 3 given its first-order transfer
%function (micro-seconds)
dz4=1247.9; % PWM dead-zone of motor 4 given its first-order transfer
% 
% g_m1=tf(k1,[tc 1]); % First-order transfer-function of motor 1
% g_m2=tf(k2,[tc 1]); % First-order transfer-function of motor 2
% g_m3=tf(k3,[tc 1]); % First-order transfer-function of motor 3
% g_m4=tf(k4,[tc 1]); % First-order transfer-function of motor 4

%vNote: If the behavior of the motors is not linear, linearization around
% an operating point is required to attain these transfer-functions.
%the motors (micro-seconds)
w0c=sqrt(g*mq/Kt);
%X0c=w0c;
Ft0=mq*g;


%% u=[T; taux; tauy; tauz];

% WTF = [ -Kt -Kt -Kt -Kt;
%          0   -lx*Kt  0  lx*Kt;
%         ly*Kt  0  -ly*Kt  0;
%         Ktm -Ktm Ktm -Ktm];   
%    T= WTF^(-1)*[Thrust; taux; tauy; tauz];

%%  u=[taux; tauy; tauz, T];

WTF = [     0   -lx*Kt  0  lx*Kt;
            -ly*Kt  0  ly*Kt  0;
            Ktm -Ktm Ktm -Ktm;
            -Kt -Kt -Kt -Kt];  
% w^2 = WTF^-1 * u
T2= WTF\[taux; tauy; tauz; Thrust];
T2Sign = sign(T2);
T=sqrt(abs(T2));
T=T2Sign.*T;

%% Conversion

    w1 = T(1);
    w2 = T(2);
    w3 = T(3);
    w4 = T(4);

== matlab function NonLinearities2/RHard/T2W ==
  data: taux input double; tauy input double; tauz input double; Thrust input double; w1 output double; w2 output double; w3 output double; w4 output double
function [w1,w2,w3,w4] = mixer(taux,tauy,tauz,Thrust)
%#codegen
%% Physical properties of the environment
g=9.81; %Acceleration of gravity (m)
rho=1.2; %Density of air (m^3.kg^-1)

%% Physical properties of the quadrotor

% Total mass of the quadrotor [Kg]
mq=0.82;
% Motor length along x-axis (m). All motors have equal sizes.
lx=28.8e-3;
% Motor length along y-axis (m)
ly=28.8e-3;
% Motor length along z-axis (m)
lz=26e-3;

% Distance from the center of gravity to the center of a motor (m).
% The quadrotor is symmetric regarding the XZ and YZ planes, so
% dcg is the same for all motors.
dcg=0.288; 


% Inflow coefficient
If = -0.3559;

% Thrust coefficient of the propeller and Power coefficient
cp=0.0743; 
ct=0.1154;

% Propeller radius (m)
rp=25.4e-3; 
% Constant value to calculate the moment provided
% by a propeller given its angular speed (kg.m^2.rad^-1)
Km=cp*4*rho*rp^5/pi()^3; 
% Constant value to calculate the thrust provided
% by a propeller given its angular speed (kg.m.rad^-1) 
%Kt=ct*4*rho*rp^4/pi()^2; 
Kt=ct*rho*rp^4*pi();
% Constant that relates thrust and moment of a propeller.
Ktm=Km/Kt;
k1=2.028; %Transfer-function gain of motor 1
k2=1.869; %Transfer-function gain of motor 2
k3=2.002; %Transfer-function gain of motor 3
k4=1.996; %Transfer-function gain of motor 4
tc=0.00436; %Time-constant of the motors (assumed equal for all motors) 0.436

dz1=1247.4; %PWM dead-zone of motor 1 given its first-order transfer
% function (micro-seconds)
dz2=1247.8; % PWM dead-zone of motor 2 given its first-order transfer
%function (micro-seconds)
dz3=1246.4; % PWM dead-zone of motor 3 given its first-order transfer
%function (micro-seconds)
dz4=1247.9; % PWM dead-zone of motor 4 given its first-order transfer
% 
% g_m1=tf(k1,[tc 1]); % First-order transfer-function of motor 1
% g_m2=tf(k2,[tc 1]); % First-order transfer-function of motor 2
% g_m3=tf(k3,[tc 1]); % First-order transfer-function of motor 3
% g_m4=tf(k4,[tc 1]); % First-order transfer-function of motor 4

%vNote: If the behavior of the motors is not linear, linearization around
% an operating point is required to attain these transfer-functions.
%the motors (micro-seconds)
w0c=sqrt(g*mq/Kt);
%X0c=w0c;
Ft0=mq*g;


%% u=[T; taux; tauy; tauz];

% WTF = [ -Kt -Kt -Kt -Kt;
%          0   -lx*Kt  0  lx*Kt;
%         ly*Kt  0  -ly*Kt  0;
%         Ktm -Ktm Ktm -Ktm];   
%    T= WTF^(-1)*[Thrust; taux; tauy; tauz];

%%  u=[taux; tauy; tauz, T];

WTF = [     0   -lx*Kt  0  lx*Kt;
            -ly*Kt  0  ly*Kt  0;
            Ktm -Ktm Ktm -Ktm;
            -Kt -Kt -Kt -Kt];  
% w^2 = WTF^-1 * u
T2= WTF\[taux; tauy; tauz; Thrust];
T2Sign = sign(T2);
T=sqrt(abs(T2));
T=T2Sign.*T;

%% Conversion

    w1 = T(1);
    w2 = T(2);
    w3 = T(3);
    w4 = T(4);

== matlab function NonLinearities2/Medium/W2T ==
  data: taux output double; tauy output double; tauz output double; Thrust output double; w1 input double; w2 input double; w3 input double; w4 input double
function [taux,tauy,tauz,Thrust] = mixerInv(w1,w2,w3,w4)
%#codegen
%% Physical properties of the environment
g=9.81; %Acceleration of gravity (m)
rho=1.2; %Density of air (m^3.kg^-1)

%% Physical properties of the quadrotor

% Total mass of the quadrotor [Kg]
mq=0.82;
% Motor length along x-axis (m). All motors have equal sizes.
lx=28.8e-3;
% Motor length along y-axis (m)
ly=28.8e-3;
% Motor length along z-axis (m)
lz=26e-3;

% Distance from the center of gravity to the center of a motor (m).
% The quadrotor is symmetric regarding the XZ and YZ planes, so
% dcg is the same for all motors.
dcg=0.288; 


% Inflow coefficient
If = -0.3559;

% Thrust coefficient of the propeller and Power coefficient
cp=0.0743; 
ct=0.1154;

% Propeller radius (m)
rp=25.4e-3; 
% Constant value to calculate the moment provided
% by a propeller given its angular speed (kg.m^2.rad^-1)
Km=cp*4*rho*rp^5/pi()^3; 
% Constant value to calculate the thrust provided
% by a propeller given its angular speed (kg.m.rad^-1) 
%Kt=ct*4*rho*rp^4/pi()^2; 
Kt=ct*rho*rp^4*pi();
% Constant that relates thrust and moment of a propeller.
Ktm=Km/Kt;
k1=2.028; %Transfer-function gain of motor 1
k2=1.869; %Transfer-function gain of motor 2
k3=2.002; %Transfer-function gain of motor 3
k4=1.996; %Transfer-function gain of motor 4
tc=0.00436; %Time-constant of the motors (assumed equal for all motors) 0.436

dz1=1247.4; %PWM dead-zone of motor 1 given its first-order transfer
% function (micro-seconds)
dz2=1247.8; % PWM dead-zone of motor 2 given its first-order transfer
%function (micro-seconds)
dz3=1246.4; % PWM dead-zone of motor 3 given its first-order transfer
%function (micro-seconds)
dz4=1247.9; % PWM dead-zone of motor 4 given its first-order transfer
% 
% g_m1=tf(k1,[tc 1]); % First-order transfer-function of motor 1
% g_m2=tf(k2,[tc 1]); % First-order transfer-function of motor 2
% g_m3=tf(k3,[tc 1]); % First-order transfer-function of motor 3
% g_m4=tf(k4,[tc 1]); % First-order transfer-function of motor 4

%vNote: If the behavior of the motors is not linear, linearization around
% an operating point is required to attain these transfer-functions.
%the motors (micro-seconds)
w0c=sqrt(g*mq/Kt);
%X0c=w0c;
Ft0=mq*g;


%% u=[T; taux; tauy; tauz];

% WTF = [ -Kt -Kt -Kt -Kt;
%          0   -lx*Kt  0  lx*Kt;
%         ly*Kt  0  -ly*Kt  0;
%         Ktm -Ktm Ktm -Ktm];   
%    T= WTF^(-1)*[Thrust; taux; tauy; tauz];

%%  u=[taux; tauy; tauz, T];

WTF = [     0   -lx*Kt  0  lx*Kt;
            -ly*Kt  0  ly*Kt  0;
            Ktm -Ktm Ktm -Ktm;
            -Kt -Kt -Kt -Kt];

w=[w1;w2;w3;w4];
wSign = sign(w);
w2 = wSign.*w.^2;
T= WTF*w2;

%% Conversion

    taux = T(1);
    tauy = T(2);
    tauz = T(3);
    Thrust = T(4);

== matlab function NonLinearities2/RHard/W2T ==
  data: taux output double; tauy output double; tauz output double; Thrust output double; w1 input double; w2 input double; w3 input double; w4 input double
function [taux,tauy,tauz,Thrust] = mixerInv(w1,w2,w3,w4)
%#codegen
%% Physical properties of the environment
g=9.81; %Acceleration of gravity (m)
rho=1.2; %Density of air (m^3.kg^-1)

%% Physical properties of the quadrotor

% Total mass of the quadrotor [Kg]
mq=0.82;
% Motor length along x-axis (m). All motors have equal sizes.
lx=28.8e-3;
% Motor length along y-axis (m)
ly=28.8e-3;
% Motor length along z-axis (m)
lz=26e-3;

% Distance from the center of gravity to the center of a motor (m).
% The quadrotor is symmetric regarding the XZ and YZ planes, so
% dcg is the same for all motors.
dcg=0.288; 


% Inflow coefficient
If = -0.3559;

% Thrust coefficient of the propeller and Power coefficient
cp=0.0743; 
ct=0.1154;

% Propeller radius (m)
rp=25.4e-3; 
% Constant value to calculate the moment provided
% by a propeller given its angular speed (kg.m^2.rad^-1)
Km=cp*4*rho*rp^5/pi()^3; 
% Constant value to calculate the thrust provided
% by a propeller given its angular speed (kg.m.rad^-1) 
%Kt=ct*4*rho*rp^4/pi()^2; 
Kt=ct*rho*rp^4*pi();
% Constant that relates thrust and moment of a propeller.
Ktm=Km/Kt;
k1=2.028; %Transfer-function gain of motor 1
k2=1.869; %Transfer-function gain of motor 2
k3=2.002; %Transfer-function gain of motor 3
k4=1.996; %Transfer-function gain of motor 4
tc=0.00436; %Time-constant of the motors (assumed equal for all motors) 0.436

dz1=1247.4; %PWM dead-zone of motor 1 given its first-order transfer
% function (micro-seconds)
dz2=1247.8; % PWM dead-zone of motor 2 given its first-order transfer
%function (micro-seconds)
dz3=1246.4; % PWM dead-zone of motor 3 given its first-order transfer
%function (micro-seconds)
dz4=1247.9; % PWM dead-zone of motor 4 given its first-order transfer
% 
% g_m1=tf(k1,[tc 1]); % First-order transfer-function of motor 1
% g_m2=tf(k2,[tc 1]); % First-order transfer-function of motor 2
% g_m3=tf(k3,[tc 1]); % First-order transfer-function of motor 3
% g_m4=tf(k4,[tc 1]); % First-order transfer-function of motor 4

%vNote: If the behavior of the motors is not linear, linearization around
% an operating point is required to attain these transfer-functions.
%the motors (micro-seconds)
w0c=sqrt(g*mq/Kt);
%X0c=w0c;
Ft0=mq*g;


%% u=[T; taux; tauy; tauz];

% WTF = [ -Kt -Kt -Kt -Kt;
%          0   -lx*Kt  0  lx*Kt;
%         ly*Kt  0  -ly*Kt  0;
%         Ktm -Ktm Ktm -Ktm];   
%    T= WTF^(-1)*[Thrust; taux; tauy; tauz];

%%  u=[taux; tauy; tauz, T];

WTF = [     0   -lx*Kt  0  lx*Kt;
            -ly*Kt  0  ly*Kt  0;
            Ktm -Ktm Ktm -Ktm;
            -Kt -Kt -Kt -Kt];

w=[w1;w2;w3;w4];
wSign = sign(w);
w2 = wSign.*w.^2;
T= WTF*w2;

%% Conversion

    taux = T(1);
    tauy = T(2);
    tauz = T(3);
    Thrust = T(4);
